simulink model "ssc_battery_management_R2012b"  (R2012b)
settings: Solver=ode15s  StartTime=0.0  StopTime=2000  FixedStep=0.1  MinStep=1e-10  RelTol=1e-5
PreLoadFcn:
  | ModelPath = fileparts(get_param(bdroot,'FileName'));
  | addpath(ModelPath);
  | 
  | ssc_battery_management_R2012b_ini
values from neighbouring files (symbols this model uses):
  AltData100AMaxCurrent =     [AlternatorTableData.mat]
  AltData100AVoltage =     [AlternatorTableData.mat]
  AltData80AMaxCurrent =     [AlternatorTableData.mat]
  AltData80AVoltage =     [AlternatorTableData.mat]
  Kt = [0.80,1.10,1.20,1.12;]    [ssc_lead_acid_battery_50Ah_ini.m]    (also in ssc_lead_acid_battery_80Ah_ini.m)
  Kt_Temps = [25 40 60 75]    [ssc_lead_acid_battery_50Ah_ini.m]    (also in ssc_lead_acid_battery_80Ah_ini.m)
  theta_f = -40    [ssc_lead_acid_battery_50Ah_ini.m]    (also in ssc_lead_acid_battery_80Ah_ini.m)
  theta_init = 25    [ssc_lead_acid_battery_50Ah_ini.m]    (also in ssc_lead_acid_battery_80Ah_ini.m)
undefined symbols (not defined in the file or in its folder): DiscIntNeverNeededParam, sigbuilder_block
undefined symbols (not defined in the file): beta, center, exponent, polyTerms, WendlandNumTerms, width
libraries: fl_lib x146, LeadAcidBattery_lib x36, nesl_utility x28, simulink x1
(part 2 of 4)

== system ssc_battery_management_R2012b/tail lamp ==
  PS Lookup Table (1D) : fl_lib/Physical Signals/Lookup Tables/PS Lookup Table (1D)  x_t=[0 voltage]  y_t=[voltage(1)/current(1) voltage./current]  interp_method=1  extrap_method=2  LocalVarLogging=[]
  PS Saturation : fl_lib/Physical Signals/Nonlinear Operators/PS Saturation  upper_limit=max(voltage./current)  lower_limit=min(voltage./current)  LocalVarLogging=[]
  Variable Resistor : fl_lib/Electrical/Electrical Elements/Variable Resistor  Rmin=0.01 Ohm  i_Log=off  v_Log=off  LocalVarNames=|i|v  LocalVarDescs=|i|v  LocalVarLogging=[0 0]
  Voltage Sensor : fl_lib/Electrical/Electrical Sensors/Voltage Sensor  i1_Log=off  v1_Log=off  LocalVarNames=|i1|v1  LocalVarDescs=|i1|v1  LocalVarLogging=[0 0]
  + : PMIOPort  Tag=PMCPort  Port=1  Side=Left
  - : PMIOPort  Tag=PMCPort  Port=2  Side=Right
  connections:
  PS Saturation/LConn1 -- PS Lookup Table (1D)/RConn1
  Voltage Sensor/RConn2 -- Variable Resistor/RConn1 -- -/RConn1
  Voltage Sensor/LConn1 -- Variable Resistor/LConn2 -- +/RConn1
  Voltage Sensor/RConn1 -- PS Lookup Table (1D)/LConn1
  PS Saturation/RConn1 -- Variable Resistor/LConn1

== system ssc_battery_management_R2012b/Alternator Variants/Alternator_100A_LUT ==
  Temp : Inport
  RPM : Inport  Port=2
  Alternator : Subsystem
  Controlled Current Source : fl_lib/Electrical/Electrical Sources/Controlled Current Source  i_Log=off  v_Log=off  LocalVarNames=|i|v  LocalVarDescs=|i|v  LocalVarLogging=[0 0]
  IC : InitialCondition  Value=14.3
  Simulink-PS Converter : nesl_utility/Simulink-PS Converter  PhysicalDomain=network_engine_domain  LeftPortType=input  RightPortType=output  SubClassName=ps_input  PseudoPeriodic=off  Frequencies=[]  NoiseDistribution=none  NoiseParameters=[]  Unit=1  AffineConversion=off  InputFilterTimeConstant=.001  UdotUserProvided=0  SimscapeFilterOrder=1  InputFiltering=off
  Voltage sensor : Subsystem
  + : PMIOPort  Tag=PMCPort  Port=1  Side=Right
  - : PMIOPort  Tag=PMCPort  Port=2  Side=Right
  tag scope: gen_current=global, gen_duty_cycle=global
  wires:
  IC/1 -> Alternator/3(Voltage)  "V"
  [gen_voltage] -> IC/1
  Alternator/1(Load Factor) -> [gen_duty_cycle]  "Load Factor"
  Alternator/2(Current) -> Simulink-PS Converter/1, [gen_current]  "Current"
  RPM/1 -> Alternator/2(RPM)  "RPM"
  Temp/1 -> Alternator/1(Temp)  "Temp"
  connections:
  Simulink-PS Converter/RConn1 -- Controlled Current Source/RConn1
  Voltage sensor/LConn1 -- +/RConn1 -- Controlled Current Source/LConn1
  -/RConn1 -- Voltage sensor/RConn1 -- Controlled Current Source/RConn2

== system ssc_battery_management_R2012b/Alternator Variants/Alternator_100A_MBC ==
  Temp : Inport
  RPM : Inport  Port=2
  Alternator : Subsystem
  Controlled Current Source : fl_lib/Electrical/Electrical Sources/Controlled Current Source  i_Log=off  v_Log=off  LocalVarNames=|i|v  LocalVarDescs=|i|v  LocalVarLogging=[0 0]
  IC : InitialCondition  Value=14.3
  Simulink-PS Converter : nesl_utility/Simulink-PS Converter  PhysicalDomain=network_engine_domain  LeftPortType=input  RightPortType=output  SubClassName=ps_input  PseudoPeriodic=off  Frequencies=[]  NoiseDistribution=none  NoiseParameters=[]  Unit=1  AffineConversion=off  InputFilterTimeConstant=.001  UdotUserProvided=0  SimscapeFilterOrder=1  InputFiltering=off
  Voltage sensor : Subsystem
  + : PMIOPort  Tag=PMCPort  Port=1  Side=Right
  - : PMIOPort  Tag=PMCPort  Port=2  Side=Right
  tag scope: gen_current=global, gen_duty_cycle=global
  wires:
  Temp/1 -> Alternator/1(Temp)  "Temp"
  RPM/1 -> Alternator/2(RPM)  "RPM"
  Alternator/2(Current) -> [gen_current], Simulink-PS Converter/1  "Current"
  Alternator/1(Load Factor) -> [gen_duty_cycle]  "Load Factor"
  [gen_voltage] -> IC/1
  IC/1 -> Alternator/3(Voltage)  "V"
  connections:
  Controlled Current Source/RConn2 -- Voltage sensor/RConn1 -- -/RConn1
  Controlled Current Source/LConn1 -- +/RConn1 -- Voltage sensor/LConn1
  Simulink-PS Converter/RConn1 -- Controlled Current Source/RConn1

== system ssc_battery_management_R2012b/Alternator Variants/Alternator_80A_LUT ==
  Temp : Inport
  RPM : Inport  Port=2
  Alternator : Subsystem
  Controlled Current Source : fl_lib/Electrical/Electrical Sources/Controlled Current Source  i_Log=off  v_Log=off  LocalVarNames=|i|v  LocalVarDescs=|i|v  LocalVarLogging=[0 0]
  IC : InitialCondition  Value=14.3
  Simulink-PS Converter : nesl_utility/Simulink-PS Converter  PhysicalDomain=network_engine_domain  LeftPortType=input  RightPortType=output  SubClassName=ps_input  PseudoPeriodic=off  Frequencies=[]  NoiseDistribution=none  NoiseParameters=[]  Unit=1  AffineConversion=off  InputFilterTimeConstant=.001  UdotUserProvided=0  SimscapeFilterOrder=1  InputFiltering=off
  Voltage sensor : Subsystem
  + : PMIOPort  Tag=PMCPort  Port=1  Side=Right
  - : PMIOPort  Tag=PMCPort  Port=2  Side=Right
  tag scope: gen_current=global, gen_duty_cycle=global
  wires:
  Temp/1 -> Alternator/1(Temp)  "Temp"
  RPM/1 -> Alternator/2(RPM)  "RPM"
  Alternator/2(Current) -> [gen_current], Simulink-PS Converter/1  "Current"
  Alternator/1(Load Factor) -> [gen_duty_cycle]  "Load Factor"
  [gen_voltage] -> IC/1
  IC/1 -> Alternator/3(Voltage)  "V"
  connections:
  Controlled Current Source/RConn2 -- Voltage sensor/RConn1 -- -/RConn1
  Controlled Current Source/LConn1 -- +/RConn1 -- Voltage sensor/LConn1
  Simulink-PS Converter/RConn1 -- Controlled Current Source/RConn1

== system ssc_battery_management_R2012b/Alternator Variants/Alternator_80A_MBC ==
  Temp : Inport
  RPM : Inport  Port=2
  Alternator : Subsystem
  Controlled Current Source : fl_lib/Electrical/Electrical Sources/Controlled Current Source  i_Log=off  v_Log=off  LocalVarNames=|i|v  LocalVarDescs=|i|v  LocalVarLogging=[0 0]
  IC : InitialCondition  Value=14.3
  Simulink-PS Converter : nesl_utility/Simulink-PS Converter  PhysicalDomain=network_engine_domain  LeftPortType=input  RightPortType=output  SubClassName=ps_input  PseudoPeriodic=off  Frequencies=[]  NoiseDistribution=none  NoiseParameters=[]  Unit=1  AffineConversion=off  InputFilterTimeConstant=.001  UdotUserProvided=0  SimscapeFilterOrder=1  InputFiltering=off
  Voltage sensor : Subsystem
  + : PMIOPort  Tag=PMCPort  Port=1  Side=Right
  - : PMIOPort  Tag=PMCPort  Port=2  Side=Right
  tag scope: gen_current=global, gen_duty_cycle=global
  wires:
  IC/1 -> Alternator/3(Voltage)  "V"
  [gen_voltage] -> IC/1
  Alternator/1(Load Factor) -> [gen_duty_cycle]  "Load Factor"
  Alternator/2(Current) -> Simulink-PS Converter/1, [gen_current]  "Current"
  RPM/1 -> Alternator/2(RPM)  "RPM"
  Temp/1 -> Alternator/1(Temp)  "Temp"
  connections:
  Simulink-PS Converter/RConn1 -- Controlled Current Source/RConn1
  Voltage sensor/LConn1 -- +/RConn1 -- Controlled Current Source/LConn1
  -/RConn1 -- Voltage sensor/RConn1 -- Controlled Current Source/RConn2

== system ssc_battery_management_R2012b/Lead-Acid Battery/Battery Cell 1 ==
  C1 : LeadAcidBattery_lib/Main Branch Capacitance, C1  Tau1=Tau1 s  Cmin=1e-5 F  i_Log=off  v_Log=off  Q_Log=off  LocalVarNames=|i|v|Q  LocalVarDescs=|Current through variable|Voltage across variable|Charge variable  LocalVarLogging=[0 0 0]
  Diode : fl_lib/Electrical/Electrical Elements/Diode  Vf=0.6 V  Ron=0.3 Ohm  Goff=1e-08 1/Ohm  i_Log=off  v_Log=off  LocalVarNames=|current|voltage|power  LocalVarDescs=|Diode current (A)|Voltage across diode (V)|Power (W)  LocalVarLogging=[0 0 0]
  Ep : fl_lib/Electrical/Electrical Sources/DC Voltage Source  v0=Ep V  i_Log=off  v_Log=off  LocalVarNames=|current|voltage|power  LocalVarDescs=|Current (A)|Voltage (V)|Power (W)  LocalVarLogging=[0 0 0]
  Main Branch Voltage Source (Em) : LeadAcidBattery_lib/Main Branch Voltage Source, Em  Em0=Emo V  Ke=Ke V/K  Kc=Kc  C0=Costar s*A  Istar=Istar A  delta=delta  Tau1=Tau1 s  Qinit=Qe_init s*A  i_Log=off  v_Log=off  Iavg_Log=off  Qe_Log=off  LocalVarNames=|i|v|cap_u|cap_t|Q|Iavg  LocalVarDescs=|Current through variable|Voltage across variable|usable battery capacity|total battery capacity|battery charge|average current given by (I/(Ts+1))  LocalVarLogging=[0 0 0 0 0 0]
  R0 : LeadAcidBattery_lib/Terminal Resistance, R0  R00=Roo Ohm  A0=Ao  i_Log=off  v_Log=off  LocalVarNames=|i|v  LocalVarDescs=|Current through variable|Voltage across variable  LocalVarLogging=[0 0]
  R1 : LeadAcidBattery_lib/Main Branch Resistance, R1  R10=R10 Ohm  DOC_min=1e-006  i_Log=off  v_Log=off  LocalVarNames=|i|v  LocalVarDescs=|Current through variable|Voltage across variable  LocalVarLogging=[0 0]
  R2 : LeadAcidBattery_lib/Main Branch Resistance, R2  R20=R20 Ohm  A21=A21  A22=A22  Istar=Istar A  i_Log=off  v_Log=off  LocalVarNames=|i|v  LocalVarDescs=|Current through variable|Voltage across variable  LocalVarLogging=[0 0]
  Rp : LeadAcidBattery_lib/Parasitic Branch Resistance, Rp  Gp0=Gpo 1/Ohm  Vp0=Vpo V  Ap=Ap  Tf=theta_f C  i_Log=off  v_Log=off  LocalVarNames=|i|v|Vavg  LocalVarDescs=|Current through variable|Voltage across variable|average voltage given by (V/(Ts+1))  LocalVarLogging=[0 0 0]
  Thermal Model : Subsystem
  H : PMIOPort  Tag=PMCPort  Port=1  Side=Right
  + : PMIOPort  Tag=PMCPort  Port=2  Side=Left
  - : PMIOPort  Tag=PMCPort  Port=3  Side=Left
  connections:
  Diode/LConn1 -- R0/RConn1 -- R2/LConn2
  R2/RConn2 -- Thermal Model/LConn1
  -/RConn1 -- Ep/RConn1 -- Main Branch Voltage Source (Em)/RConn1
  Thermal Model/RConn1 -- Main Branch Voltage Source (Em)/RConn3
  Diode/RConn1 -- Rp/LConn1
  Ep/LConn1 -- Rp/RConn2
  Thermal Model/LConn2 -- H/RConn1
  R2/LConn1 -- Main Branch Voltage Source (Em)/LConn1 -- R0/LConn1
  R1/LConn2 -- C1/LConn1
  R1/LConn1 -- C1/LConn2 -- R2/RConn1
  Main Branch Voltage Source (Em)/LConn3 -- C1/RConn1 -- R1/RConn2
  Main Branch Voltage Source (Em)/LConn2 -- R1/RConn1
  R0/LConn2 -- +/RConn1
  Thermal Model/RConn2 -- Main Branch Voltage Source (Em)/RConn2 -- Rp/RConn1

== system ssc_battery_management_R2012b/Lead-Acid Battery/Battery Cell 2 ==
  C1 : LeadAcidBattery_lib/Main Branch Capacitance, C1  Tau1=Tau1 s  Cmin=1e-5 F  i_Log=off  v_Log=off  Q_Log=off  LocalVarNames=|i|v|Q  LocalVarDescs=|Current through variable|Voltage across variable|Charge variable  LocalVarLogging=[0 0 0]
  Diode : fl_lib/Electrical/Electrical Elements/Diode  Vf=0.6 V  Ron=0.3 Ohm  Goff=1e-08 1/Ohm  i_Log=off  v_Log=off  LocalVarNames=|current|voltage|power  LocalVarDescs=|Diode current (A)|Voltage across diode (V)|Power (W)  LocalVarLogging=[0 0 0]
  Ep : fl_lib/Electrical/Electrical Sources/DC Voltage Source  v0=Ep V  i_Log=off  v_Log=off  LocalVarNames=|current|voltage|power  LocalVarDescs=|Current (A)|Voltage (V)|Power (W)  LocalVarLogging=[0 0 0]
  Main Branch Voltage Source (Em) : LeadAcidBattery_lib/Main Branch Voltage Source, Em  Em0=Emo V  Ke=Ke V/K  Kc=Kc  C0=Costar s*A  Istar=Istar A  delta=delta  Tau1=Tau1 s  Qinit=Qe_init s*A  i_Log=off  v_Log=off  Iavg_Log=off  Qe_Log=off  LocalVarNames=|i|v|cap_u|cap_t|Q|Iavg  LocalVarDescs=|Current through variable|Voltage across variable|usable battery capacity|total battery capacity|battery charge|average current given by (I/(Ts+1))  LocalVarLogging=[0 0 0 0 0 0]
  R0 : LeadAcidBattery_lib/Terminal Resistance, R0  R00=Roo Ohm  A0=Ao  i_Log=off  v_Log=off  LocalVarNames=|i|v  LocalVarDescs=|Current through variable|Voltage across variable  LocalVarLogging=[0 0]
  R1 : LeadAcidBattery_lib/Main Branch Resistance, R1  R10=R10 Ohm  DOC_min=1e-006  i_Log=off  v_Log=off  LocalVarNames=|i|v  LocalVarDescs=|Current through variable|Voltage across variable  LocalVarLogging=[0 0]
  R2 : LeadAcidBattery_lib/Main Branch Resistance, R2  R20=R20 Ohm  A21=A21  A22=A22  Istar=Istar A  i_Log=off  v_Log=off  LocalVarNames=|i|v  LocalVarDescs=|Current through variable|Voltage across variable  LocalVarLogging=[0 0]
  Rp : LeadAcidBattery_lib/Parasitic Branch Resistance, Rp  Gp0=Gpo 1/Ohm  Vp0=Vpo V  Ap=Ap  Tf=theta_f C  i_Log=off  v_Log=off  LocalVarNames=|i|v|Vavg  LocalVarDescs=|Current through variable|Voltage across variable|average voltage given by (V/(Ts+1))  LocalVarLogging=[0 0 0]
  Thermal Model : Subsystem
  H : PMIOPort  Tag=PMCPort  Port=1  Side=Right
  + : PMIOPort  Tag=PMCPort  Port=2  Side=Left
  - : PMIOPort  Tag=PMCPort  Port=3  Side=Left
  connections:
  Rp/RConn1 -- Main Branch Voltage Source (Em)/RConn2 -- Thermal Model/RConn2
  R0/LConn2 -- +/RConn1
  Main Branch Voltage Source (Em)/LConn2 -- R1/RConn1
  R1/RConn2 -- C1/RConn1 -- Main Branch Voltage Source (Em)/LConn3
  R2/RConn1 -- C1/LConn2 -- R1/LConn1
  R1/LConn2 -- C1/LConn1
  R0/LConn1 -- Main Branch Voltage Source (Em)/LConn1 -- R2/LConn1
  Thermal Model/LConn2 -- H/RConn1
  Ep/LConn1 -- Rp/RConn2
  Diode/RConn1 -- Rp/LConn1
  Thermal Model/RConn1 -- Main Branch Voltage Source (Em)/RConn3
  Main Branch Voltage Source (Em)/RConn1 -- Ep/RConn1 -- -/RConn1
  R2/RConn2 -- Thermal Model/LConn1
  R2/LConn2 -- R0/RConn1 -- Diode/LConn1

== system ssc_battery_management_R2012b/Lead-Acid Battery/Battery Cell 3 ==
  C1 : LeadAcidBattery_lib/Main Branch Capacitance, C1  Tau1=Tau1 s  Cmin=1e-5 F  i_Log=off  v_Log=off  Q_Log=off  LocalVarNames=|i|v|Q  LocalVarDescs=|Current through variable|Voltage across variable|Charge variable  LocalVarLogging=[0 0 0]
  Diode : fl_lib/Electrical/Electrical Elements/Diode  Vf=0.6 V  Ron=0.3 Ohm  Goff=1e-08 1/Ohm  i_Log=off  v_Log=off  LocalVarNames=|current|voltage|power  LocalVarDescs=|Diode current (A)|Voltage across diode (V)|Power (W)  LocalVarLogging=[0 0 0]
  Ep : fl_lib/Electrical/Electrical Sources/DC Voltage Source  v0=Ep V  i_Log=off  v_Log=off  LocalVarNames=|current|voltage|power  LocalVarDescs=|Current (A)|Voltage (V)|Power (W)  LocalVarLogging=[0 0 0]
  Main Branch Voltage Source (Em) : LeadAcidBattery_lib/Main Branch Voltage Source, Em  Em0=Emo V  Ke=Ke V/K  Kc=Kc  C0=Costar s*A  Istar=Istar A  delta=delta  Tau1=Tau1 s  Qinit=Qe_init s*A  i_Log=off  v_Log=off  Iavg_Log=off  Qe_Log=off  LocalVarNames=|i|v|cap_u|cap_t|Q|Iavg  LocalVarDescs=|Current through variable|Voltage across variable|usable battery capacity|total battery capacity|battery charge|average current given by (I/(Ts+1))  LocalVarLogging=[0 0 0 0 0 0]
  R0 : LeadAcidBattery_lib/Terminal Resistance, R0  R00=Roo Ohm  A0=Ao  i_Log=off  v_Log=off  LocalVarNames=|i|v  LocalVarDescs=|Current through variable|Voltage across variable  LocalVarLogging=[0 0]
  R1 : LeadAcidBattery_lib/Main Branch Resistance, R1  R10=R10 Ohm  DOC_min=1e-006  i_Log=off  v_Log=off  LocalVarNames=|i|v  LocalVarDescs=|Current through variable|Voltage across variable  LocalVarLogging=[0 0]
  R2 : LeadAcidBattery_lib/Main Branch Resistance, R2  R20=R20 Ohm  A21=A21  A22=A22  Istar=Istar A  i_Log=off  v_Log=off  LocalVarNames=|i|v  LocalVarDescs=|Current through variable|Voltage across variable  LocalVarLogging=[0 0]
  Rp : LeadAcidBattery_lib/Parasitic Branch Resistance, Rp  Gp0=Gpo 1/Ohm  Vp0=Vpo V  Ap=Ap  Tf=theta_f C  i_Log=off  v_Log=off  LocalVarNames=|i|v|Vavg  LocalVarDescs=|Current through variable|Voltage across variable|average voltage given by (V/(Ts+1))  LocalVarLogging=[0 0 0]
  Thermal Model : Subsystem
  H : PMIOPort  Tag=PMCPort  Port=1  Side=Right
  + : PMIOPort  Tag=PMCPort  Port=2  Side=Left
  - : PMIOPort  Tag=PMCPort  Port=3  Side=Left
  connections:
  Rp/RConn1 -- Main Branch Voltage Source (Em)/RConn2 -- Thermal Model/RConn2
  R0/LConn2 -- +/RConn1
  Main Branch Voltage Source (Em)/LConn2 -- R1/RConn1
  R1/RConn2 -- C1/RConn1 -- Main Branch Voltage Source (Em)/LConn3
  R2/RConn1 -- C1/LConn2 -- R1/LConn1
  R1/LConn2 -- C1/LConn1
  R0/LConn1 -- Main Branch Voltage Source (Em)/LConn1 -- R2/LConn1
  Thermal Model/LConn2 -- H/RConn1
  Ep/LConn1 -- Rp/RConn2
  Diode/RConn1 -- Rp/LConn1
  Thermal Model/RConn1 -- Main Branch Voltage Source (Em)/RConn3
  Main Branch Voltage Source (Em)/RConn1 -- Ep/RConn1 -- -/RConn1
  R2/RConn2 -- Thermal Model/LConn1
  R2/LConn2 -- R0/RConn1 -- Diode/LConn1

== system ssc_battery_management_R2012b/Lead-Acid Battery/Battery Cell 4 ==
  C1 : LeadAcidBattery_lib/Main Branch Capacitance, C1  Tau1=Tau1 s  Cmin=1e-5 F  i_Log=off  v_Log=off  Q_Log=off  LocalVarNames=|i|v|Q  LocalVarDescs=|Current through variable|Voltage across variable|Charge variable  LocalVarLogging=[0 0 0]
  Diode : fl_lib/Electrical/Electrical Elements/Diode  Vf=0.6 V  Ron=0.3 Ohm  Goff=1e-08 1/Ohm  i_Log=off  v_Log=off  LocalVarNames=|current|voltage|power  LocalVarDescs=|Diode current (A)|Voltage across diode (V)|Power (W)  LocalVarLogging=[0 0 0]
  Ep : fl_lib/Electrical/Electrical Sources/DC Voltage Source  v0=Ep V  i_Log=off  v_Log=off  LocalVarNames=|current|voltage|power  LocalVarDescs=|Current (A)|Voltage (V)|Power (W)  LocalVarLogging=[0 0 0]
  Main Branch Voltage Source (Em) : LeadAcidBattery_lib/Main Branch Voltage Source, Em  Em0=Emo V  Ke=Ke V/K  Kc=Kc  C0=Costar s*A  Istar=Istar A  delta=delta  Tau1=Tau1 s  Qinit=Qe_init s*A  i_Log=off  v_Log=off  Iavg_Log=off  Qe_Log=off  LocalVarNames=|i|v|cap_u|cap_t|Q|Iavg  LocalVarDescs=|Current through variable|Voltage across variable|usable battery capacity|total battery capacity|battery charge|average current given by (I/(Ts+1))  LocalVarLogging=[0 0 0 0 0 0]
  R0 : LeadAcidBattery_lib/Terminal Resistance, R0  R00=Roo Ohm  A0=Ao  i_Log=off  v_Log=off  LocalVarNames=|i|v  LocalVarDescs=|Current through variable|Voltage across variable  LocalVarLogging=[0 0]
  R1 : LeadAcidBattery_lib/Main Branch Resistance, R1  R10=R10 Ohm  DOC_min=1e-006  i_Log=off  v_Log=off  LocalVarNames=|i|v  LocalVarDescs=|Current through variable|Voltage across variable  LocalVarLogging=[0 0]
  R2 : LeadAcidBattery_lib/Main Branch Resistance, R2  R20=R20 Ohm  A21=A21  A22=A22  Istar=Istar A  i_Log=off  v_Log=off  LocalVarNames=|i|v  LocalVarDescs=|Current through variable|Voltage across variable  LocalVarLogging=[0 0]
  Rp : LeadAcidBattery_lib/Parasitic Branch Resistance, Rp  Gp0=Gpo 1/Ohm  Vp0=Vpo V  Ap=Ap  Tf=theta_f C  i_Log=off  v_Log=off  LocalVarNames=|i|v|Vavg  LocalVarDescs=|Current through variable|Voltage across variable|average voltage given by (V/(Ts+1))  LocalVarLogging=[0 0 0]
  Thermal Model : Subsystem
  H : PMIOPort  Tag=PMCPort  Port=1  Side=Right
  + : PMIOPort  Tag=PMCPort  Port=2  Side=Left
  - : PMIOPort  Tag=PMCPort  Port=3  Side=Left
  connections:
  Rp/RConn1 -- Main Branch Voltage Source (Em)/RConn2 -- Thermal Model/RConn2
  R0/LConn2 -- +/RConn1
  Main Branch Voltage Source (Em)/LConn2 -- R1/RConn1
  R1/RConn2 -- C1/RConn1 -- Main Branch Voltage Source (Em)/LConn3
  R2/RConn1 -- C1/LConn2 -- R1/LConn1
  R1/LConn2 -- C1/LConn1
  R0/LConn1 -- Main Branch Voltage Source (Em)/LConn1 -- R2/LConn1
  Thermal Model/LConn2 -- H/RConn1
  Ep/LConn1 -- Rp/RConn2
  Diode/RConn1 -- Rp/LConn1
  Thermal Model/RConn1 -- Main Branch Voltage Source (Em)/RConn3
  Main Branch Voltage Source (Em)/RConn1 -- Ep/RConn1 -- -/RConn1
  R2/RConn2 -- Thermal Model/LConn1
  R2/LConn2 -- R0/RConn1 -- Diode/LConn1

== system ssc_battery_management_R2012b/Lead-Acid Battery/Battery Cell 5 ==
  C1 : LeadAcidBattery_lib/Main Branch Capacitance, C1  Tau1=Tau1 s  Cmin=1e-5 F  i_Log=off  v_Log=off  Q_Log=off  LocalVarNames=|i|v|Q  LocalVarDescs=|Current through variable|Voltage across variable|Charge variable  LocalVarLogging=[0 0 0]
  Diode : fl_lib/Electrical/Electrical Elements/Diode  Vf=0.6 V  Ron=0.3 Ohm  Goff=1e-08 1/Ohm  i_Log=off  v_Log=off  LocalVarNames=|current|voltage|power  LocalVarDescs=|Diode current (A)|Voltage across diode (V)|Power (W)  LocalVarLogging=[0 0 0]
  Ep : fl_lib/Electrical/Electrical Sources/DC Voltage Source  v0=Ep V  i_Log=off  v_Log=off  LocalVarNames=|current|voltage|power  LocalVarDescs=|Current (A)|Voltage (V)|Power (W)  LocalVarLogging=[0 0 0]
  Main Branch Voltage Source (Em) : LeadAcidBattery_lib/Main Branch Voltage Source, Em  Em0=Emo V  Ke=Ke V/K  Kc=Kc  C0=Costar s*A  Istar=Istar A  delta=delta  Tau1=Tau1 s  Qinit=Qe_init s*A  i_Log=off  v_Log=off  Iavg_Log=off  Qe_Log=off  LocalVarNames=|i|v|cap_u|cap_t|Q|Iavg  LocalVarDescs=|Current through variable|Voltage across variable|usable battery capacity|total battery capacity|battery charge|average current given by (I/(Ts+1))  LocalVarLogging=[0 0 0 0 0 0]
  R0 : LeadAcidBattery_lib/Terminal Resistance, R0  R00=Roo Ohm  A0=Ao  i_Log=off  v_Log=off  LocalVarNames=|i|v  LocalVarDescs=|Current through variable|Voltage across variable  LocalVarLogging=[0 0]
  R1 : LeadAcidBattery_lib/Main Branch Resistance, R1  R10=R10 Ohm  DOC_min=1e-006  i_Log=off  v_Log=off  LocalVarNames=|i|v  LocalVarDescs=|Current through variable|Voltage across variable  LocalVarLogging=[0 0]
  R2 : LeadAcidBattery_lib/Main Branch Resistance, R2  R20=R20 Ohm  A21=A21  A22=A22  Istar=Istar A  i_Log=off  v_Log=off  LocalVarNames=|i|v  LocalVarDescs=|Current through variable|Voltage across variable  LocalVarLogging=[0 0]
  Rp : LeadAcidBattery_lib/Parasitic Branch Resistance, Rp  Gp0=Gpo 1/Ohm  Vp0=Vpo V  Ap=Ap  Tf=theta_f C  i_Log=off  v_Log=off  LocalVarNames=|i|v|Vavg  LocalVarDescs=|Current through variable|Voltage across variable|average voltage given by (V/(Ts+1))  LocalVarLogging=[0 0 0]
  Thermal Model : Subsystem
  H : PMIOPort  Tag=PMCPort  Port=1  Side=Right
  + : PMIOPort  Tag=PMCPort  Port=2  Side=Left
  - : PMIOPort  Tag=PMCPort  Port=3  Side=Left
  connections:
  Rp/RConn1 -- Main Branch Voltage Source (Em)/RConn2 -- Thermal Model/RConn2
  R0/LConn2 -- +/RConn1
  Main Branch Voltage Source (Em)/LConn2 -- R1/RConn1
  R1/RConn2 -- C1/RConn1 -- Main Branch Voltage Source (Em)/LConn3
  R2/RConn1 -- C1/LConn2 -- R1/LConn1
  R1/LConn2 -- C1/LConn1
  R0/LConn1 -- Main Branch Voltage Source (Em)/LConn1 -- R2/LConn1
  Thermal Model/LConn2 -- H/RConn1
  Ep/LConn1 -- Rp/RConn2
  Diode/RConn1 -- Rp/LConn1
  Thermal Model/RConn1 -- Main Branch Voltage Source (Em)/RConn3
  Main Branch Voltage Source (Em)/RConn1 -- Ep/RConn1 -- -/RConn1
  R2/RConn2 -- Thermal Model/LConn1
  R2/LConn2 -- R0/RConn1 -- Diode/LConn1

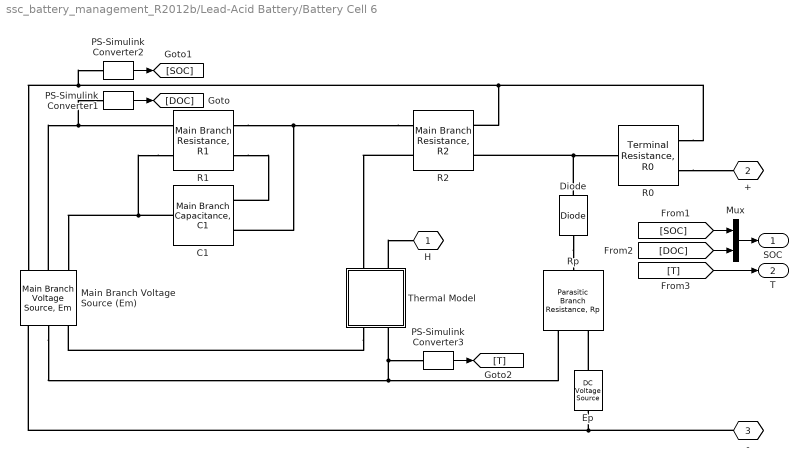
== system ssc_battery_management_R2012b/Lead-Acid Battery/Battery Cell 6 ==
  C1 : LeadAcidBattery_lib/Main Branch Capacitance, C1  Tau1=Tau1 s  Cmin=1e-5 F  i_Log=off  v_Log=off  Q_Log=off  LocalVarNames=|i|v|Q  LocalVarDescs=|Current through variable|Voltage across variable|Charge variable  LocalVarLogging=[0 0 0]
  Diode : fl_lib/Electrical/Electrical Elements/Diode  Vf=0.6 V  Ron=0.3 Ohm  Goff=1e-08 1/Ohm  i_Log=off  v_Log=off  LocalVarNames=|current|voltage|power  LocalVarDescs=|Diode current (A)|Voltage across diode (V)|Power (W)  LocalVarLogging=[0 0 0]
  Ep : fl_lib/Electrical/Electrical Sources/DC Voltage Source  v0=Ep V  i_Log=off  v_Log=off  LocalVarNames=|current|voltage|power  LocalVarDescs=|Current (A)|Voltage (V)|Power (W)  LocalVarLogging=[0 0 0]
  Main Branch Voltage Source (Em) : LeadAcidBattery_lib/Main Branch Voltage Source, Em  Em0=Emo V  Ke=Ke V/K  Kc=Kc  C0=Costar s*A  Istar=Istar A  delta=delta  Tau1=Tau1 s  Qinit=Qe_init s*A  i_Log=off  v_Log=off  Iavg_Log=off  Qe_Log=off  LocalVarNames=|i|v|cap_u|cap_t|Q|Iavg  LocalVarDescs=|Current through variable|Voltage across variable|usable battery capacity|total battery capacity|battery charge|average current given by (I/(Ts+1))  LocalVarLogging=[0 0 0 0 0 0]
  Mux : Mux  Inputs=2
  PS-Simulink Converter1 : nesl_utility/PS-Simulink Converter  PhysicalDomain=network_engine_domain  LeftPortType=input  RightPortType=output  SubClassName=ps_output  PseudoPeriodic=off  Frequencies=[]  Unit=1  AffineConversion=off
  PS-Simulink Converter2 : nesl_utility/PS-Simulink Converter  PhysicalDomain=network_engine_domain  LeftPortType=input  RightPortType=output  SubClassName=ps_output  PseudoPeriodic=off  Frequencies=[]  Unit=1  AffineConversion=off
  PS-Simulink Converter3 : nesl_utility/PS-Simulink Converter  PhysicalDomain=network_engine_domain  LeftPortType=input  RightPortType=output  SubClassName=ps_output  PseudoPeriodic=off  Frequencies=[]  Unit=1  AffineConversion=off
  R0 : LeadAcidBattery_lib/Terminal Resistance, R0  R00=Roo Ohm  A0=Ao  i_Log=off  v_Log=off  LocalVarNames=|i|v  LocalVarDescs=|Current through variable|Voltage across variable  LocalVarLogging=[0 0]
  R1 : LeadAcidBattery_lib/Main Branch Resistance, R1  R10=R10 Ohm  DOC_min=1e-006  i_Log=off  v_Log=off  LocalVarNames=|i|v  LocalVarDescs=|Current through variable|Voltage across variable  LocalVarLogging=[0 0]
  R2 : LeadAcidBattery_lib/Main Branch Resistance, R2  R20=R20 Ohm  A21=A21  A22=A22  Istar=Istar A  i_Log=off  v_Log=off  LocalVarNames=|i|v  LocalVarDescs=|Current through variable|Voltage across variable  LocalVarLogging=[0 0]
  Rp : LeadAcidBattery_lib/Parasitic Branch Resistance, Rp  Gp0=Gpo 1/Ohm  Vp0=Vpo V  Ap=Ap  Tf=theta_f C  i_Log=off  v_Log=off  LocalVarNames=|i|v|Vavg  LocalVarDescs=|Current through variable|Voltage across variable|average voltage given by (V/(Ts+1))  LocalVarLogging=[0 0 0]
  Thermal Model : Subsystem
  H : PMIOPort  Tag=PMCPort  Port=1  Side=Right
  + : PMIOPort  Tag=PMCPort  Port=2  Side=Left
  - : PMIOPort  Tag=PMCPort  Port=3  Side=Left
  SOC : Outport
  T : Outport  Port=2
  wires:
  Mux/1 -> SOC/1
  [SOC] -> Mux/1
  [DOC] -> Mux/2
  [T] -> T/1
  PS-Simulink Converter1/1 -> [DOC]
  PS-Simulink Converter2/1 -> [SOC]
  PS-Simulink Converter3/1 -> [T]
  connections:
  Rp/RConn1 -- Main Branch Voltage Source (Em)/RConn2 -- Thermal Model/RConn2 -- PS-Simulink Converter3/LConn1
  R0/LConn2 -- +/RConn1
  Main Branch Voltage Source (Em)/LConn2 -- R1/RConn1 -- PS-Simulink Converter1/LConn1
  R1/RConn2 -- C1/RConn1 -- Main Branch Voltage Source (Em)/LConn3
  R2/RConn1 -- C1/LConn2 -- R1/LConn1
  R1/LConn2 -- C1/LConn1
  R0/LConn1 -- Main Branch Voltage Source (Em)/LConn1 -- PS-Simulink Converter2/LConn1 -- R2/LConn1
  Thermal Model/LConn2 -- H/RConn1
  Ep/LConn1 -- Rp/RConn2
  Diode/RConn1 -- Rp/LConn1
  Thermal Model/RConn1 -- Main Branch Voltage Source (Em)/RConn3
  Main Branch Voltage Source (Em)/RConn1 -- Ep/RConn1 -- -/RConn1
  R2/RConn2 -- Thermal Model/LConn1
  R2/LConn2 -- R0/RConn1 -- Diode/LConn1

== system ssc_battery_management_R2012b/Lead-Acid Battery/Current Sensor ==
  Current Sensor : fl_lib/Electrical/Electrical Sensors/Current Sensor  i1_Log=off  v1_Log=off  LocalVarNames=|i1|v1  LocalVarDescs=|i1|v1  LocalVarLogging=[]
  PS-Simulink : nesl_utility/PS-Simulink Converter  PhysicalDomain=network_engine_domain  LeftPortType=input  RightPortType=output  SubClassName=ps_output  PseudoPeriodic=off  Frequencies=[]  Unit=A  AffineConversion=off
  + : PMIOPort  Port=1  Side=Left
  - : PMIOPort  Port=2  Side=Right
  tag scope: batt_current=global
  wires:
  PS-Simulink/1 -> [batt_current]
  connections:
  -/RConn1 -- Current Sensor/RConn2
  Current Sensor/LConn1 -- +/RConn1
  Current Sensor/RConn1 -- PS-Simulink/LConn1

== system ssc_battery_management_R2012b/Lead-Acid Battery/Stop if SOC <= 0 ==
  Compare To Zero : simulink/Logic and Bit Operations/Compare To Zero  relop=<=  OutDataTypeStr=boolean  ZeroCross=off
  Stop Simulation : Stop
  wires:
  Compare To Zero/1 -> Stop Simulation/1
  [SOC] -> Compare To Zero/1

== system ssc_battery_management_R2012b/Lead-Acid Battery/Voltage Sensor ==
  PS-Simulink Converter : nesl_utility/PS-Simulink Converter  PhysicalDomain=network_engine_domain  LeftPortType=input  RightPortType=output  SubClassName=ps_output  PseudoPeriodic=off  Frequencies=[]  Unit=V  AffineConversion=off
  Voltage Sensor : fl_lib/Electrical/Electrical Sensors/Voltage Sensor  i1_Log=off  v1_Log=off  LocalVarNames=|i1|v1  LocalVarDescs=|i1|v1  LocalVarLogging=[]
  + : PMIOPort  Port=1  Side=Left
  - : PMIOPort  Port=2  Side=Right
  tag scope: batt_voltage=global
  wires:
  PS-Simulink Converter/1 -> [batt_voltage]
  connections:
  Voltage Sensor/RConn1 -- PS-Simulink Converter/LConn1
  +/RConn1 -- Voltage Sensor/LConn1
  -/RConn1 -- Voltage Sensor/RConn2

== system ssc_battery_management_R2012b/Alternator Variants/Alternator_100A_LUT/Alternator ==
  Temp : Inport
  RPM : Inport  Port=2
  Voltage : Inport  Port=3
  100A_Max_Current : Lookup_n-D  NumberOfTableDimensions=3  BreakpointsForDimension1=AltData100AMaxCurrent.RPM  BreakpointsForDimension2=AltData100AMaxCurrent.Voltage  BreakpointsForDimension3=AltData100AMaxCurrent.Temp  Table=AltData100AMaxCurrent.Current  InputSameDT=on
  100A_Voltage : Lookup_n-D  NumberOfTableDimensions=3  BreakpointsForDimension1=AltData100AVoltage.RPM  BreakpointsForDimension2=AltData100AVoltage.Current  BreakpointsForDimension3=AltData100AVoltage.Temp  Table=AltData100AVoltage.Voltage  InputSameDT=on
  Product : Product  Inputs=/*  SaturateOnIntegerOverflow=on  OutDataTypeStr=Inherit: Same as first input
  Regulate Voltage : Subsystem
  Saturation1 : Saturate  UpperLimit=inf  LowerLimit=1e-9  ZeroCross=off
  Saturation2 : Saturate  UpperLimit=1  LowerLimit=0  ZeroCross=off
  Saturation3 : Saturate  UpperLimit=15  LowerLimit=13  ZeroCross=off
  Sum : Sum  Inputs=-+|  SaturateOnIntegerOverflow=on
  Load Factor : Outport
  Current : Outport  Port=2
  wires:
  Saturation2/1 -> Load Factor/1
  Saturation1/1 -> Regulate Voltage/1(Max_Current), Product/1  "Max Current"
  Saturation3/1 -> Sum/2  "V_reg"
  Regulate Voltage/1(i) -> Current/1, Product/2, 100A_Voltage/2  "Current"
  Voltage/1 -> Sum/1, 100A_Max_Current/2  "V"
  100A_Max_Current/1 -> Saturation1/1  "Max Current"
  Sum/1 -> Regulate Voltage/2(V error)  "V error"
  100A_Voltage/1 -> Saturation3/1
  RPM/1 -> 100A_Max_Current/1, 100A_Voltage/1  "RPM"
  Temp/1 -> 100A_Max_Current/3, 100A_Voltage/3  "Temp"
  Product/1 -> Saturation2/1

== system ssc_battery_management_R2012b/Alternator Variants/Alternator_100A_LUT/Voltage sensor ==
  PS-Simulink Converter : nesl_utility/PS-Simulink Converter  PhysicalDomain=network_engine_domain  LeftPortType=input  RightPortType=output  SubClassName=ps_output  PseudoPeriodic=off  Frequencies=[]  Unit=V  AffineConversion=off
  Voltage Sensor : fl_lib/Electrical/Electrical Sensors/Voltage Sensor  i1_Log=off  v1_Log=off  LocalVarNames=|i1|v1  LocalVarDescs=|i1|v1  LocalVarLogging=[]
  + : PMIOPort  Port=1  Side=Left
  - : PMIOPort  Port=2  Side=Right
  tag scope: gen_voltage=global
  wires:
  PS-Simulink Converter/1 -> [gen_voltage]
  connections:
  -/RConn1 -- Voltage Sensor/RConn2
  +/RConn1 -- Voltage Sensor/LConn1
  Voltage Sensor/RConn1 -- PS-Simulink Converter/LConn1

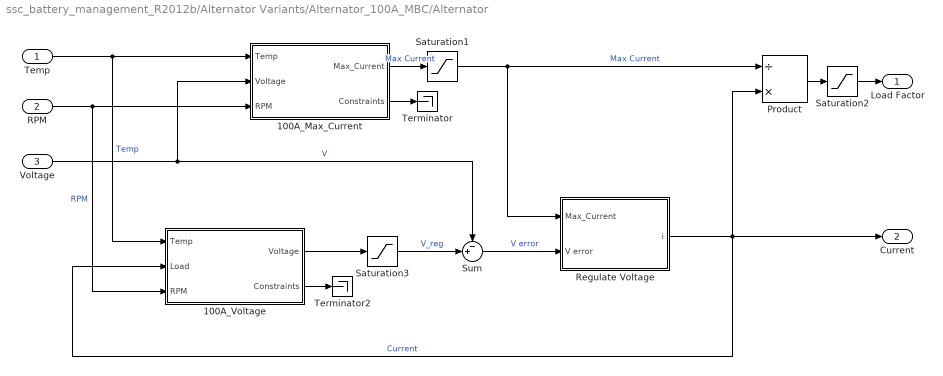
== system ssc_battery_management_R2012b/Alternator Variants/Alternator_100A_MBC/Alternator ==
  Temp : Inport
  RPM : Inport  Port=2
  Voltage : Inport  Port=3
  100A_Max_Current : Subsystem
  100A_Voltage : Subsystem
  Product : Product  Inputs=/*  SaturateOnIntegerOverflow=on  OutDataTypeStr=Inherit: Same as first input
  Regulate Voltage : Subsystem
  Saturation1 : Saturate  UpperLimit=inf  LowerLimit=1e-9  ZeroCross=off
  Saturation2 : Saturate  UpperLimit=1  LowerLimit=0  ZeroCross=off
  Saturation3 : Saturate  UpperLimit=15  LowerLimit=13  ZeroCross=off
  Sum : Sum  Inputs=-+|  SaturateOnIntegerOverflow=on
  Terminator : Terminator
  Terminator2 : Terminator
  Load Factor : Outport
  Current : Outport  Port=2
  wires:
  100A_Max_Current/2(Constraints) -> Terminator/1
  Product/1 -> Saturation2/1
  Temp/1 -> 100A_Voltage/1(Temp), 100A_Max_Current/1(Temp)  "Temp"
  RPM/1 -> 100A_Voltage/3(RPM), 100A_Max_Current/3(RPM)  "RPM"
  100A_Voltage/2(Constraints) -> Terminator2/1
  100A_Voltage/1(Voltage) -> Saturation3/1
  Sum/1 -> Regulate Voltage/2(V error)  "V error"
  100A_Max_Current/1(Max_Current) -> Saturation1/1  "Max Current"
  Voltage/1 -> Sum/1, 100A_Max_Current/2(Voltage)  "V"
  Regulate Voltage/1(i) -> Product/2, Current/1, 100A_Voltage/2(Load)  "Current"
  Saturation3/1 -> Sum/2  "V_reg"
  Saturation1/1 -> Product/1, Regulate Voltage/1(Max_Current)  "Max Current"
  Saturation2/1 -> Load Factor/1

== system ssc_battery_management_R2012b/Alternator Variants/Alternator_100A_MBC/Voltage sensor ==
  PS-Simulink Converter : nesl_utility/PS-Simulink Converter  PhysicalDomain=network_engine_domain  LeftPortType=input  RightPortType=output  SubClassName=ps_output  PseudoPeriodic=off  Frequencies=[]  Unit=V  AffineConversion=off
  Voltage Sensor : fl_lib/Electrical/Electrical Sensors/Voltage Sensor  i1_Log=off  v1_Log=off  LocalVarNames=|i1|v1  LocalVarDescs=|i1|v1  LocalVarLogging=[]
  + : PMIOPort  Port=1  Side=Left
  - : PMIOPort  Port=2  Side=Right
  tag scope: gen_voltage=global
  wires:
  PS-Simulink Converter/1 -> [gen_voltage]
  connections:
  Voltage Sensor/RConn1 -- PS-Simulink Converter/LConn1
  +/RConn1 -- Voltage Sensor/LConn1
  -/RConn1 -- Voltage Sensor/RConn2

== system ssc_battery_management_R2012b/Alternator Variants/Alternator_80A_LUT/Alternator ==
  Temp : Inport
  RPM : Inport  Port=2
  Voltage : Inport  Port=3
  80A_Max_Current : Lookup_n-D  NumberOfTableDimensions=3  BreakpointsForDimension1=AltData80AMaxCurrent.RPM  BreakpointsForDimension2=AltData80AMaxCurrent.Voltage  BreakpointsForDimension3=AltData80AMaxCurrent.Temp  Table=AltData80AMaxCurrent.Current  InputSameDT=on
  80A_Voltage : Lookup_n-D  NumberOfTableDimensions=3  BreakpointsForDimension1=AltData80AVoltage.RPM  BreakpointsForDimension2=AltData80AVoltage.Current  BreakpointsForDimension3=AltData80AVoltage.Temp  Table=AltData80AVoltage.Voltage  InputSameDT=on
  Product : Product  Inputs=/*  SaturateOnIntegerOverflow=on  OutDataTypeStr=Inherit: Same as first input
  Regulate Voltage : Subsystem
  Saturation1 : Saturate  UpperLimit=inf  LowerLimit=1e-9  ZeroCross=off
  Saturation2 : Saturate  UpperLimit=1  LowerLimit=0  ZeroCross=off
  Saturation3 : Saturate  UpperLimit=15  LowerLimit=13  ZeroCross=off
  Sum : Sum  Inputs=-+|  SaturateOnIntegerOverflow=on
  Load Factor : Outport
  Current : Outport  Port=2
  wires:
  Saturation2/1 -> Load Factor/1
  Product/1 -> Saturation2/1
  Temp/1 -> 80A_Voltage/3, 80A_Max_Current/3  "Temp"
  RPM/1 -> 80A_Voltage/1, 80A_Max_Current/1  "RPM"
  80A_Voltage/1 -> Saturation3/1
  Sum/1 -> Regulate Voltage/2(V error)  "V error"
  80A_Max_Current/1 -> Saturation1/1  "Max Current"
  Voltage/1 -> Sum/1, 80A_Max_Current/2  "V"
  Regulate Voltage/1(i) -> Product/2, Current/1, 80A_Voltage/2  "Current"
  Saturation3/1 -> Sum/2  "V_reg"
  Saturation1/1 -> Product/1, Regulate Voltage/1(Max_Current)  "Max Current"

== system ssc_battery_management_R2012b/Alternator Variants/Alternator_80A_LUT/Voltage sensor ==
  PS-Simulink Converter : nesl_utility/PS-Simulink Converter  PhysicalDomain=network_engine_domain  LeftPortType=input  RightPortType=output  SubClassName=ps_output  PseudoPeriodic=off  Frequencies=[]  Unit=V  AffineConversion=off
  Voltage Sensor : fl_lib/Electrical/Electrical Sensors/Voltage Sensor  i1_Log=off  v1_Log=off  LocalVarNames=|i1|v1  LocalVarDescs=|i1|v1  LocalVarLogging=[]
  + : PMIOPort  Port=1  Side=Left
  - : PMIOPort  Port=2  Side=Right
  tag scope: gen_voltage=global
  wires:
  PS-Simulink Converter/1 -> [gen_voltage]
  connections:
  Voltage Sensor/RConn1 -- PS-Simulink Converter/LConn1
  +/RConn1 -- Voltage Sensor/LConn1
  -/RConn1 -- Voltage Sensor/RConn2

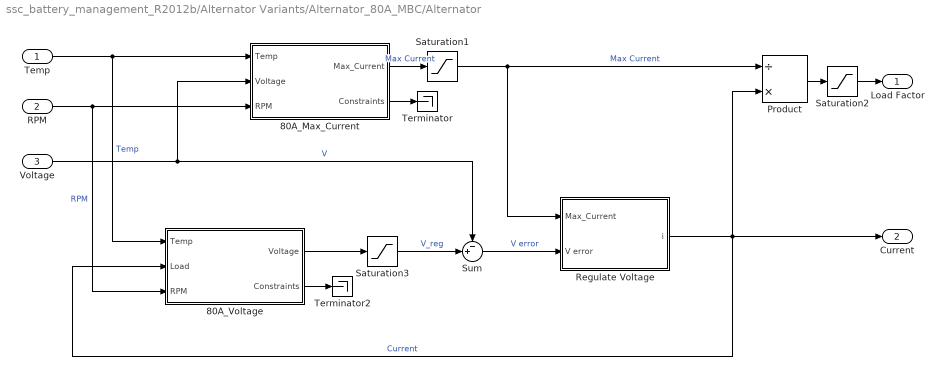
== system ssc_battery_management_R2012b/Alternator Variants/Alternator_80A_MBC/Alternator ==
  Temp : Inport
  RPM : Inport  Port=2
  Voltage : Inport  Port=3
  80A_Max_Current : Subsystem
  80A_Voltage : Subsystem
  Product : Product  Inputs=/*  SaturateOnIntegerOverflow=on  OutDataTypeStr=Inherit: Same as first input
  Regulate Voltage : Subsystem
  Saturation1 : Saturate  UpperLimit=inf  LowerLimit=1e-9  ZeroCross=off
  Saturation2 : Saturate  UpperLimit=1  LowerLimit=0  ZeroCross=off
  Saturation3 : Saturate  UpperLimit=15  LowerLimit=13  ZeroCross=off
  Sum : Sum  Inputs=-+|  SaturateOnIntegerOverflow=on
  Terminator : Terminator
  Terminator2 : Terminator
  Load Factor : Outport
  Current : Outport  Port=2
  wires:
  Saturation1/1 -> Regulate Voltage/1(Max_Current), Product/1  "Max Current"
  Saturation3/1 -> Sum/2  "V_reg"
  Regulate Voltage/1(i) -> Current/1, Product/2, 80A_Voltage/2(Load)  "Current"
  Voltage/1 -> Sum/1, 80A_Max_Current/2(Voltage)  "V"
  80A_Max_Current/1(Max_Current) -> Saturation1/1  "Max Current"
  Sum/1 -> Regulate Voltage/2(V error)  "V error"
  80A_Voltage/1(Voltage) -> Saturation3/1
  80A_Voltage/2(Constraints) -> Terminator2/1
  RPM/1 -> 80A_Max_Current/3(RPM), 80A_Voltage/3(RPM)  "RPM"
  Temp/1 -> 80A_Max_Current/1(Temp), 80A_Voltage/1(Temp)  "Temp"
  Product/1 -> Saturation2/1
  80A_Max_Current/2(Constraints) -> Terminator/1
  Saturation2/1 -> Load Factor/1

== system ssc_battery_management_R2012b/Alternator Variants/Alternator_80A_MBC/Voltage sensor ==
  PS-Simulink Converter : nesl_utility/PS-Simulink Converter  PhysicalDomain=network_engine_domain  LeftPortType=input  RightPortType=output  SubClassName=ps_output  PseudoPeriodic=off  Frequencies=[]  Unit=V  AffineConversion=off
  Voltage Sensor : fl_lib/Electrical/Electrical Sensors/Voltage Sensor  i1_Log=off  v1_Log=off  LocalVarNames=|i1|v1  LocalVarDescs=|i1|v1  LocalVarLogging=[]
  + : PMIOPort  Port=1  Side=Left
  - : PMIOPort  Port=2  Side=Right
  tag scope: gen_voltage=global
  wires:
  PS-Simulink Converter/1 -> [gen_voltage]
  connections:
  -/RConn1 -- Voltage Sensor/RConn2
  +/RConn1 -- Voltage Sensor/LConn1
  Voltage Sensor/RConn1 -- PS-Simulink Converter/LConn1

== system ssc_battery_management_R2012b/Lead-Acid Battery/Battery Cell 1/Thermal Model ==
  Battery thermal mass : fl_lib/Thermal/Thermal Elements/Thermal Mass  mass=1 kg  sp_heat=Ctheta J/kg/K  init_temp=theta_init+273 K  Q_Log=off  LocalVarNames=|heat_flow|temperature  LocalVarDescs=|Heat flow (J/s)|Mass temperature (K)  LocalVarLogging=[0 0]
  Ideal Temperature Sensor : fl_lib/Thermal/Thermal Sensors/Ideal Temperature Sensor  Qs_Log=off  Ts_Log=off  LocalVarNames=|Qs|Ts  LocalVarDescs=|Qs|Ts  LocalVarLogging=[]
  Ideal Heat Flow Source : fl_lib/Thermal/Thermal Sources/Ideal Heat Flow Source  Q_Log=off  T_Log=off  LocalVarNames=|heat_flow|T_differential  LocalVarDescs=|Heat flow through the source (J/s)|Temperature differential across the source (K)  LocalVarLogging=[0 0]
  Kt as a function of temperature : fl_lib/Physical Signals/Lookup Tables/PS Lookup Table (1D)  x_t=[theta_f, Kt_Temps]+273  y_t=[0 Kt]  interp_method=1  extrap_method=1  LocalVarLogging=[]
  Thermal Reference1 : fl_lib/Thermal/Thermal Elements/Thermal Reference  Q_Log=off  LocalVarNames=|Q  LocalVarDescs=|Q  LocalVarLogging=[]
  Thermal Reference2 : fl_lib/Thermal/Thermal Elements/Thermal Reference  Q_Log=off  LocalVarNames=|Q  LocalVarDescs=|Q  LocalVarLogging=[]
  Ps : PMIOPort  Tag=PMCPort  Port=1  Side=Left
  H : PMIOPort  Tag=PMCPort  Port=2  Side=Left
  Kt : PMIOPort  Tag=PMCPort  Port=3  Side=Right
  T : PMIOPort  Tag=PMCPort  Port=4  Side=Right
  connections:
  Ideal Heat Flow Source/RConn1 -- Ps/RConn1
  Kt/RConn1 -- Kt as a function of temperature/RConn1
  Battery thermal mass/LConn1 -- Ideal Heat Flow Source/LConn1 -- Ideal Temperature Sensor/LConn1 -- H/RConn1
  Thermal Reference1/LConn1 -- Ideal Heat Flow Source/RConn2
  T/RConn1 -- Kt as a function of temperature/LConn1 -- Ideal Temperature Sensor/RConn2
  Ideal Temperature Sensor/RConn1 -- Thermal Reference2/LConn1

== system ssc_battery_management_R2012b/Lead-Acid Battery/Battery Cell 2/Thermal Model ==
  Battery thermal mass : fl_lib/Thermal/Thermal Elements/Thermal Mass  mass=1 kg  sp_heat=Ctheta J/kg/K  init_temp=theta_init+273 K  Q_Log=off  LocalVarNames=|heat_flow|temperature  LocalVarDescs=|Heat flow (J/s)|Mass temperature (K)  LocalVarLogging=[0 0]
  Ideal Temperature Sensor : fl_lib/Thermal/Thermal Sensors/Ideal Temperature Sensor  Qs_Log=off  Ts_Log=off  LocalVarNames=|Qs|Ts  LocalVarDescs=|Qs|Ts  LocalVarLogging=[]
  Ideal Heat Flow Source : fl_lib/Thermal/Thermal Sources/Ideal Heat Flow Source  Q_Log=off  T_Log=off  LocalVarNames=|heat_flow|T_differential  LocalVarDescs=|Heat flow through the source (J/s)|Temperature differential across the source (K)  LocalVarLogging=[0 0]
  Kt as a function of temperature : fl_lib/Physical Signals/Lookup Tables/PS Lookup Table (1D)  x_t=[theta_f, Kt_Temps]+273  y_t=[0 Kt]  interp_method=1  extrap_method=1  LocalVarLogging=[]
  Thermal Reference1 : fl_lib/Thermal/Thermal Elements/Thermal Reference  Q_Log=off  LocalVarNames=|Q  LocalVarDescs=|Q  LocalVarLogging=[]
  Thermal Reference2 : fl_lib/Thermal/Thermal Elements/Thermal Reference  Q_Log=off  LocalVarNames=|Q  LocalVarDescs=|Q  LocalVarLogging=[]
  Ps : PMIOPort  Tag=PMCPort  Port=1  Side=Left
  H : PMIOPort  Tag=PMCPort  Port=2  Side=Left
  Kt : PMIOPort  Tag=PMCPort  Port=3  Side=Right
  T : PMIOPort  Tag=PMCPort  Port=4  Side=Right
  connections:
  Ideal Temperature Sensor/RConn1 -- Thermal Reference2/LConn1
  Ideal Temperature Sensor/RConn2 -- Kt as a function of temperature/LConn1 -- T/RConn1
  Thermal Reference1/LConn1 -- Ideal Heat Flow Source/RConn2
  H/RConn1 -- Ideal Temperature Sensor/LConn1 -- Ideal Heat Flow Source/LConn1 -- Battery thermal mass/LConn1
  Kt/RConn1 -- Kt as a function of temperature/RConn1
  Ideal Heat Flow Source/RConn1 -- Ps/RConn1

== system ssc_battery_management_R2012b/Lead-Acid Battery/Battery Cell 3/Thermal Model ==
  Battery thermal mass : fl_lib/Thermal/Thermal Elements/Thermal Mass  mass=1 kg  sp_heat=Ctheta J/kg/K  init_temp=theta_init+273 K  Q_Log=off  LocalVarNames=|heat_flow|temperature  LocalVarDescs=|Heat flow (J/s)|Mass temperature (K)  LocalVarLogging=[0 0]
  Ideal Temperature Sensor : fl_lib/Thermal/Thermal Sensors/Ideal Temperature Sensor  Qs_Log=off  Ts_Log=off  LocalVarNames=|Qs|Ts  LocalVarDescs=|Qs|Ts  LocalVarLogging=[]
  Ideal Heat Flow Source : fl_lib/Thermal/Thermal Sources/Ideal Heat Flow Source  Q_Log=off  T_Log=off  LocalVarNames=|heat_flow|T_differential  LocalVarDescs=|Heat flow through the source (J/s)|Temperature differential across the source (K)  LocalVarLogging=[0 0]
  Kt as a function of temperature : fl_lib/Physical Signals/Lookup Tables/PS Lookup Table (1D)  x_t=[theta_f, Kt_Temps]+273  y_t=[0 Kt]  interp_method=1  extrap_method=1  LocalVarLogging=[]
  Thermal Reference1 : fl_lib/Thermal/Thermal Elements/Thermal Reference  Q_Log=off  LocalVarNames=|Q  LocalVarDescs=|Q  LocalVarLogging=[]
  Thermal Reference2 : fl_lib/Thermal/Thermal Elements/Thermal Reference  Q_Log=off  LocalVarNames=|Q  LocalVarDescs=|Q  LocalVarLogging=[]
  Ps : PMIOPort  Tag=PMCPort  Port=1  Side=Left
  H : PMIOPort  Tag=PMCPort  Port=2  Side=Left
  Kt : PMIOPort  Tag=PMCPort  Port=3  Side=Right
  T : PMIOPort  Tag=PMCPort  Port=4  Side=Right
  connections:
  Ideal Temperature Sensor/RConn1 -- Thermal Reference2/LConn1
  Ideal Temperature Sensor/RConn2 -- Kt as a function of temperature/LConn1 -- T/RConn1
  Thermal Reference1/LConn1 -- Ideal Heat Flow Source/RConn2
  H/RConn1 -- Ideal Temperature Sensor/LConn1 -- Ideal Heat Flow Source/LConn1 -- Battery thermal mass/LConn1
  Kt/RConn1 -- Kt as a function of temperature/RConn1
  Ideal Heat Flow Source/RConn1 -- Ps/RConn1

== system ssc_battery_management_R2012b/Lead-Acid Battery/Battery Cell 4/Thermal Model ==
  Battery thermal mass : fl_lib/Thermal/Thermal Elements/Thermal Mass  mass=1 kg  sp_heat=Ctheta J/kg/K  init_temp=theta_init+273 K  Q_Log=off  LocalVarNames=|heat_flow|temperature  LocalVarDescs=|Heat flow (J/s)|Mass temperature (K)  LocalVarLogging=[0 0]
  Ideal Temperature Sensor : fl_lib/Thermal/Thermal Sensors/Ideal Temperature Sensor  Qs_Log=off  Ts_Log=off  LocalVarNames=|Qs|Ts  LocalVarDescs=|Qs|Ts  LocalVarLogging=[]
  Ideal Heat Flow Source : fl_lib/Thermal/Thermal Sources/Ideal Heat Flow Source  Q_Log=off  T_Log=off  LocalVarNames=|heat_flow|T_differential  LocalVarDescs=|Heat flow through the source (J/s)|Temperature differential across the source (K)  LocalVarLogging=[0 0]
  Kt as a function of temperature : fl_lib/Physical Signals/Lookup Tables/PS Lookup Table (1D)  x_t=[theta_f, Kt_Temps]+273  y_t=[0 Kt]  interp_method=1  extrap_method=1  LocalVarLogging=[]
  Thermal Reference1 : fl_lib/Thermal/Thermal Elements/Thermal Reference  Q_Log=off  LocalVarNames=|Q  LocalVarDescs=|Q  LocalVarLogging=[]
  Thermal Reference2 : fl_lib/Thermal/Thermal Elements/Thermal Reference  Q_Log=off  LocalVarNames=|Q  LocalVarDescs=|Q  LocalVarLogging=[]
  Ps : PMIOPort  Tag=PMCPort  Port=1  Side=Left
  H : PMIOPort  Tag=PMCPort  Port=2  Side=Left
  Kt : PMIOPort  Tag=PMCPort  Port=3  Side=Right
  T : PMIOPort  Tag=PMCPort  Port=4  Side=Right
  connections:
  Ideal Temperature Sensor/RConn1 -- Thermal Reference2/LConn1
  Ideal Temperature Sensor/RConn2 -- Kt as a function of temperature/LConn1 -- T/RConn1
  Thermal Reference1/LConn1 -- Ideal Heat Flow Source/RConn2
  H/RConn1 -- Ideal Temperature Sensor/LConn1 -- Ideal Heat Flow Source/LConn1 -- Battery thermal mass/LConn1
  Kt/RConn1 -- Kt as a function of temperature/RConn1
  Ideal Heat Flow Source/RConn1 -- Ps/RConn1

== system ssc_battery_management_R2012b/Lead-Acid Battery/Battery Cell 5/Thermal Model ==
  Battery thermal mass : fl_lib/Thermal/Thermal Elements/Thermal Mass  mass=1 kg  sp_heat=Ctheta J/kg/K  init_temp=theta_init+273 K  Q_Log=off  LocalVarNames=|heat_flow|temperature  LocalVarDescs=|Heat flow (J/s)|Mass temperature (K)  LocalVarLogging=[0 0]
  Ideal Temperature Sensor : fl_lib/Thermal/Thermal Sensors/Ideal Temperature Sensor  Qs_Log=off  Ts_Log=off  LocalVarNames=|Qs|Ts  LocalVarDescs=|Qs|Ts  LocalVarLogging=[]
  Ideal Heat Flow Source : fl_lib/Thermal/Thermal Sources/Ideal Heat Flow Source  Q_Log=off  T_Log=off  LocalVarNames=|heat_flow|T_differential  LocalVarDescs=|Heat flow through the source (J/s)|Temperature differential across the source (K)  LocalVarLogging=[0 0]
  Kt as a function of temperature : fl_lib/Physical Signals/Lookup Tables/PS Lookup Table (1D)  x_t=[theta_f, Kt_Temps]+273  y_t=[0 Kt]  interp_method=1  extrap_method=1  LocalVarLogging=[]
  Thermal Reference1 : fl_lib/Thermal/Thermal Elements/Thermal Reference  Q_Log=off  LocalVarNames=|Q  LocalVarDescs=|Q  LocalVarLogging=[]
  Thermal Reference2 : fl_lib/Thermal/Thermal Elements/Thermal Reference  Q_Log=off  LocalVarNames=|Q  LocalVarDescs=|Q  LocalVarLogging=[]
  Ps : PMIOPort  Tag=PMCPort  Port=1  Side=Left
  H : PMIOPort  Tag=PMCPort  Port=2  Side=Left
  Kt : PMIOPort  Tag=PMCPort  Port=3  Side=Right
  T : PMIOPort  Tag=PMCPort  Port=4  Side=Right
  connections:
  Ideal Temperature Sensor/RConn1 -- Thermal Reference2/LConn1
  Ideal Temperature Sensor/RConn2 -- Kt as a function of temperature/LConn1 -- T/RConn1
  Thermal Reference1/LConn1 -- Ideal Heat Flow Source/RConn2
  H/RConn1 -- Ideal Temperature Sensor/LConn1 -- Ideal Heat Flow Source/LConn1 -- Battery thermal mass/LConn1
  Kt/RConn1 -- Kt as a function of temperature/RConn1
  Ideal Heat Flow Source/RConn1 -- Ps/RConn1

== system ssc_battery_management_R2012b/Lead-Acid Battery/Battery Cell 6/Thermal Model ==
  Battery thermal mass : fl_lib/Thermal/Thermal Elements/Thermal Mass  mass=1 kg  sp_heat=Ctheta J/kg/K  init_temp=theta_init+273 K  Q_Log=off  LocalVarNames=|heat_flow|temperature  LocalVarDescs=|Heat flow (J/s)|Mass temperature (K)  LocalVarLogging=[0 0]
  Ideal Temperature Sensor : fl_lib/Thermal/Thermal Sensors/Ideal Temperature Sensor  Qs_Log=off  Ts_Log=off  LocalVarNames=|Qs|Ts  LocalVarDescs=|Qs|Ts  LocalVarLogging=[]
  Ideal Heat Flow Source : fl_lib/Thermal/Thermal Sources/Ideal Heat Flow Source  Q_Log=off  T_Log=off  LocalVarNames=|heat_flow|T_differential  LocalVarDescs=|Heat flow through the source (J/s)|Temperature differential across the source (K)  LocalVarLogging=[0 0]
  Kt as a function of temperature : fl_lib/Physical Signals/Lookup Tables/PS Lookup Table (1D)  x_t=[theta_f, Kt_Temps]+273  y_t=[0 Kt]  interp_method=1  extrap_method=1  LocalVarLogging=[]
  Thermal Reference1 : fl_lib/Thermal/Thermal Elements/Thermal Reference  Q_Log=off  LocalVarNames=|Q  LocalVarDescs=|Q  LocalVarLogging=[]
  Thermal Reference2 : fl_lib/Thermal/Thermal Elements/Thermal Reference  Q_Log=off  LocalVarNames=|Q  LocalVarDescs=|Q  LocalVarLogging=[]
  Ps : PMIOPort  Tag=PMCPort  Port=1  Side=Left
  H : PMIOPort  Tag=PMCPort  Port=2  Side=Left
  Kt : PMIOPort  Tag=PMCPort  Port=3  Side=Right
  T : PMIOPort  Tag=PMCPort  Port=4  Side=Right
  connections:
  Ideal Temperature Sensor/RConn1 -- Thermal Reference2/LConn1
  Ideal Temperature Sensor/RConn2 -- Kt as a function of temperature/LConn1 -- T/RConn1
  Thermal Reference1/LConn1 -- Ideal Heat Flow Source/RConn2
  H/RConn1 -- Ideal Temperature Sensor/LConn1 -- Ideal Heat Flow Source/LConn1 -- Battery thermal mass/LConn1
  Kt/RConn1 -- Kt as a function of temperature/RConn1
  Ideal Heat Flow Source/RConn1 -- Ps/RConn1
